simulink model "bug_apostrophe"  (Simulink 8.0)
settings: Solver=ode45  StartTime=0.0  StopTime=10.0  RelTol=1e-3
undefined symbols (not defined in the file): g_bias, g_sat, g_sen, g_sf_cc
settings Model: Creator=ldnascim  LastModifiedBy=ldnascim

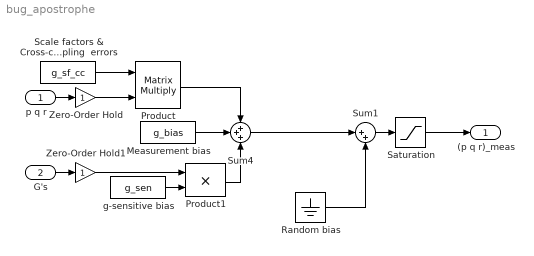
== system bug_apostrophe ==
  p q r : Inport  PortDimensions=3
  G's : Inport  Port=2  PortDimensions=3
  Measurement bias : Constant  Value=g_bias
  Product : Product  Multiplication=Matrix(*)  SaturateOnIntegerOverflow=on  OutDataTypeStr=Inherit: Same as first input
  Product1 : Product  SaturateOnIntegerOverflow=on  OutDataTypeStr=Inherit: Same as first input
  Random bias : Ground
  Saturation : Saturate  UpperLimit=g_sat(4:6)  LowerLimit=g_sat(1:3)
  "Scale factors & Cross-coupling  errors " : Constant  Value=g_sf_cc
  Sum1 : Sum  Inputs=|++  SaturateOnIntegerOverflow=on
  Sum4 : Sum  Inputs=+++  SaturateOnIntegerOverflow=on
  Zero-Order Hold : Gain  SaturateOnIntegerOverflow=on  OutDataTypeStr=Inherit: Same as input  ParamDataTypeStr=Inherit: Same as input
  Zero-Order Hold1 : Gain  SaturateOnIntegerOverflow=on  OutDataTypeStr=Inherit: Same as input  ParamDataTypeStr=Inherit: Same as input
  g-sensitive bias : Constant  Value=g_sen
  (p q r)_meas : Outport
  wires:
  Measurement bias/1 -> Sum4/2
  Product/1 -> Sum4/1
  Sum4/1 -> Sum1/1
  "Scale factors & Cross-coupling  errors "/1 -> Product/1
  Random bias/1 -> Sum1/2
  Saturation/1 -> (p q r)_meas/1
  p q r/1 -> Zero-Order Hold/1
  g-sensitive bias/1 -> Product1/2
  Sum1/1 -> Saturation/1
  G's/1 -> Zero-Order Hold1/1
  Product1/1 -> Sum4/3
  Zero-Order Hold/1 -> Product/2
  Zero-Order Hold1/1 -> Product1/1
